simulink model "nonop_quadcopter_package_delivery"  (R2024b)
settings: Solver=VariableStepAuto  StartTime=0.0  StopTime=timespot_spl(end)+2  FixedStep=0.01  MaxStep=1e-2  RelTol=1e-3  AbsTol=1e-3
model workspace (MATLAB code in the model file):
  | load('xy_data_membrane.mat');
undefined symbols (not defined in the file): air_rho, battery_capacity, drone_leg, filtD_altitude, filtD_attitude, filtD_motor, filtD_position, filtD_yaw, filtM_altitude, filtM_attitude, filtM_position, filtM_yaw, filtSpd_motor, kd_altitude, kd_attitude, kd_motor, kd_position, kd_yaw, ki_altitude, ki_attitude, ki_motor, ki_position, ki_yaw, kp_altitude, kp_attitude, kp_motor, kp_position, kp_yaw, limit_altitude, limit_attitude, limit_motor, limit_yaw, planedepth, pos2attitude, propeller, qc_motor, qd_area, qd_drag, spline_data, spline_yaw, timespot_spl, waypoints, wind_speed, X, Y, Z
libraries: sm_lib x73, fl_lib x49, nesl_utility x41, slpidlib x9, batt_lib x4, BatteryEstimators x4, ee_lib x4, quadcopter_library x4, batteryecm_lib x1
(part 4 of 5)

== system nonop_quadcopter_package_delivery/Quadcopter/Electrical/Control2 ==
  ref : Inport
  meas : Inport  Port=2
  Add : Sum  Inputs=+-
  Control : slpidlib/PID Controller  Controller=PID  Form=Parallel  TimeDomain=Continuous-time  UseExternalTs=off  SampleTime=-1  IntegratorMethod=Forward Euler  FilterMethod=Forward Euler  ControllerParametersSource=internal  P=kp  I=ki  UseKiTs=off  D=kd  UseExternalDerivativeSource=off  N=f_deriv  UseFilter=on  TunerSelectOption=Transfer Function Based (PID Tuner App)  ZeroCross=off  InitialConditionSource=internal  InitialConditionForIntegrator=0  InitialConditionForFilter=0  DifferentiatorICPrevScaledInput=0  ExternalReset=none  TrackingMode=off  Kt=1  LimitOutput=on  SatLimitsSource=internal  UpperSaturationLimit=max_trq_cmd  LowerSaturationLimit=-max_trq_cmd  LinearizeAsGain=on  AntiWindupMode=clamping  Kb=1  LimitIntegrator=off  UpperIntegratorSaturationLimit=inf  LowerIntegratorSaturationLimit=-inf  POutMin=[]  POutMax=[]  IOutMin=[]  IOutMax=[]  DOutMin=[]  DOutMax=[]  NOutMin=[]  NOutMax=[]  SumOutMin=[]  SumOutMax=[]  SaturationOutMin=[]  SaturationOutMax=[]  PParamMin=[]  PParamMax=[]  IParamMin=[]  IParamMax=[]  DParamMin=[]  DParamMax=[]  NParamMin=[]  NParamMax=[]  KbParamMin=[]  KbParamMax=[]  KtParamMin=[]  KtParamMax=[]  KbOutMin=[]  KbOutMax=[]  KtOutMin=[]  KtOutMax=[]  IntegratorOutMin=[]  IntegratorOutMax=[]  FilterOutMin=[]  FilterOutMax=[]  SumI1OutMin=[]  SumI1OutMax=[]  SumI2OutMin=[]  SumI2OutMax=[]  SumI3OutMin=[]  SumI3OutMax=[]  SumI4OutMin=[]  SumI4OutMax=[]  SumDOutMin=[]  SumDOutMax=[]  DifferentiatorOutMin=[]  DifferentiatorOutMax=[]  FilterDiffOutCoefMin=[]  FilterDiffOutCoefMax=[]  ReciprocalOutMin=[]  ReciprocalOutMax=[]  SumDenOutMin=[]  SumDenOutMax=[]  SumNumOutMin=[]  SumNumOutMax=[]  DivideOutMin=[]  DivideOutMax=[]  UdiffTsProdOutMin=[]  UdiffTsProdOutMax=[]  NTsProdOutMin=[]  NTsProdOutMax=[]  UintegralTsProdOutMin=[]  UintegralTsProdOutMax=[]  UngainTsProdOutMin=[]  UngainTsProdOutMax=[]  ClampingZeroOutDataTypeStr=Inherit: Inherit via back propagation  ClampingZeroOutMin=[]  ClampingZeroOutMax=[]  FilterDenConstantOutDataTypeStr=Inherit: Inherit via back propagation  FilterDenConstantOutMin=[]  FilterDenConstantOutMax=[]  PCopyOutDataTypeStr=Inherit: Inherit via back propagation  PCopyOutMin=[]  PCopyOutMax=[]  NCopyOutDataTypeStr=Inherit: Inherit via back propagation  NCopyOutMin=[]  NCopyOutMax=[]  IntegratorContinuousStateAttributes=''  IntegratorStateMustResolveToSignalObject=off  IntegratorRTWStateStorageClass=Auto  FilterContinuousStateAttributes=''  FilterStateMustResolveToSignalObject=off  FilterRTWStateStorageClass=Auto  ParallelPVariant=InternalParameters  IdealPVariant=Disabled  IVariant=InternalParameters  DVariant=InternalParameters  IntegratorVariant=Continuous  SatVariant=Enabled  AWVariant=ContClampingParallel  PCopyVariant=Disabled  TRVariant=Disabled  FdbkBlocksVariant=Forward  IdealPFdbkVariant=Disabled  SatFdbkVariant=Disabled  DerivativeFilterVariant=ContFilter  NVariant=InternalParameters  NCopyVariant=Disabled  FilterICVariant=InternalICsFilter  IntegratorICVariant=InternalICs  ExternalResetVariant=Disabled  TRSumVariant=Passthrough  SumFdbkVariant=Disabled  SumVariant=Sum_PID  TsampFilterVariant=InternalTs  TsampNgainVariant=Passthrough  TsampIntegralVariant=Disabled_SignalSpec  ExternalSaturationOutDataTypeStr=Inherit: Same as second input  DerivativeSourceVariant=ErrorSignal  PreIntVariant=InternalPreInt
  Mux : Mux  Inputs=2
  Scope : Scope  NumInputPorts=3
  Transfer Fcn1 : TransferFcn  Denominator=[f_spd 1]
  torque : Outport
  wires:
  Control/1 -> torque/1, Scope/3  "torque"
  ref/1 -> Add/1, Mux/1
  Add/1 -> Scope/2, Control/1  "error"
  Mux/1 -> Scope/1
  meas/1 -> Transfer Fcn1/1
  Transfer Fcn1/1 -> Add/2, Mux/2

== system nonop_quadcopter_package_delivery/Quadcopter/Electrical/Control3 ==
  ref : Inport
  meas : Inport  Port=2
  Add : Sum  Inputs=+-
  Control : slpidlib/PID Controller  Controller=PID  Form=Parallel  TimeDomain=Continuous-time  UseExternalTs=off  SampleTime=-1  IntegratorMethod=Forward Euler  FilterMethod=Forward Euler  ControllerParametersSource=internal  P=kp  I=ki  UseKiTs=off  D=kd  UseExternalDerivativeSource=off  N=f_deriv  UseFilter=on  TunerSelectOption=Transfer Function Based (PID Tuner App)  ZeroCross=off  InitialConditionSource=internal  InitialConditionForIntegrator=0  InitialConditionForFilter=0  DifferentiatorICPrevScaledInput=0  ExternalReset=none  TrackingMode=off  Kt=1  LimitOutput=on  SatLimitsSource=internal  UpperSaturationLimit=max_trq_cmd  LowerSaturationLimit=-max_trq_cmd  LinearizeAsGain=on  AntiWindupMode=clamping  Kb=1  LimitIntegrator=off  UpperIntegratorSaturationLimit=inf  LowerIntegratorSaturationLimit=-inf  POutMin=[]  POutMax=[]  IOutMin=[]  IOutMax=[]  DOutMin=[]  DOutMax=[]  NOutMin=[]  NOutMax=[]  SumOutMin=[]  SumOutMax=[]  SaturationOutMin=[]  SaturationOutMax=[]  PParamMin=[]  PParamMax=[]  IParamMin=[]  IParamMax=[]  DParamMin=[]  DParamMax=[]  NParamMin=[]  NParamMax=[]  KbParamMin=[]  KbParamMax=[]  KtParamMin=[]  KtParamMax=[]  KbOutMin=[]  KbOutMax=[]  KtOutMin=[]  KtOutMax=[]  IntegratorOutMin=[]  IntegratorOutMax=[]  FilterOutMin=[]  FilterOutMax=[]  SumI1OutMin=[]  SumI1OutMax=[]  SumI2OutMin=[]  SumI2OutMax=[]  SumI3OutMin=[]  SumI3OutMax=[]  SumI4OutMin=[]  SumI4OutMax=[]  SumDOutMin=[]  SumDOutMax=[]  DifferentiatorOutMin=[]  DifferentiatorOutMax=[]  FilterDiffOutCoefMin=[]  FilterDiffOutCoefMax=[]  ReciprocalOutMin=[]  ReciprocalOutMax=[]  SumDenOutMin=[]  SumDenOutMax=[]  SumNumOutMin=[]  SumNumOutMax=[]  DivideOutMin=[]  DivideOutMax=[]  UdiffTsProdOutMin=[]  UdiffTsProdOutMax=[]  NTsProdOutMin=[]  NTsProdOutMax=[]  UintegralTsProdOutMin=[]  UintegralTsProdOutMax=[]  UngainTsProdOutMin=[]  UngainTsProdOutMax=[]  ClampingZeroOutDataTypeStr=Inherit: Inherit via back propagation  ClampingZeroOutMin=[]  ClampingZeroOutMax=[]  FilterDenConstantOutDataTypeStr=Inherit: Inherit via back propagation  FilterDenConstantOutMin=[]  FilterDenConstantOutMax=[]  PCopyOutDataTypeStr=Inherit: Inherit via back propagation  PCopyOutMin=[]  PCopyOutMax=[]  NCopyOutDataTypeStr=Inherit: Inherit via back propagation  NCopyOutMin=[]  NCopyOutMax=[]  IntegratorContinuousStateAttributes=''  IntegratorStateMustResolveToSignalObject=off  IntegratorRTWStateStorageClass=Auto  FilterContinuousStateAttributes=''  FilterStateMustResolveToSignalObject=off  FilterRTWStateStorageClass=Auto  ParallelPVariant=InternalParameters  IdealPVariant=Disabled  IVariant=InternalParameters  DVariant=InternalParameters  IntegratorVariant=Continuous  SatVariant=Enabled  AWVariant=ContClampingParallel  PCopyVariant=Disabled  TRVariant=Disabled  FdbkBlocksVariant=Forward  IdealPFdbkVariant=Disabled  SatFdbkVariant=Disabled  DerivativeFilterVariant=ContFilter  NVariant=InternalParameters  NCopyVariant=Disabled  FilterICVariant=InternalICsFilter  IntegratorICVariant=InternalICs  ExternalResetVariant=Disabled  TRSumVariant=Passthrough  SumFdbkVariant=Disabled  SumVariant=Sum_PID  TsampFilterVariant=InternalTs  TsampNgainVariant=Passthrough  TsampIntegralVariant=Disabled_SignalSpec  ExternalSaturationOutDataTypeStr=Inherit: Same as second input  DerivativeSourceVariant=ErrorSignal  PreIntVariant=InternalPreInt
  Mux : Mux  Inputs=2
  Scope : Scope  NumInputPorts=3
  Transfer Fcn1 : TransferFcn  Denominator=[f_spd 1]
  torque : Outport
  wires:
  Control/1 -> torque/1, Scope/3  "torque"
  ref/1 -> Add/1, Mux/1
  Add/1 -> Scope/2, Control/1  "error"
  Mux/1 -> Scope/1
  meas/1 -> Transfer Fcn1/1
  Transfer Fcn1/1 -> Add/2, Mux/2

== system nonop_quadcopter_package_delivery/Quadcopter/Electrical/Control4 ==
  ref : Inport
  meas : Inport  Port=2
  Add : Sum  Inputs=+-
  Control : slpidlib/PID Controller  Controller=PID  Form=Parallel  TimeDomain=Continuous-time  UseExternalTs=off  SampleTime=-1  IntegratorMethod=Forward Euler  FilterMethod=Forward Euler  ControllerParametersSource=internal  P=kp  I=ki  UseKiTs=off  D=kd  UseExternalDerivativeSource=off  N=f_deriv  UseFilter=on  TunerSelectOption=Transfer Function Based (PID Tuner App)  ZeroCross=off  InitialConditionSource=internal  InitialConditionForIntegrator=0  InitialConditionForFilter=0  DifferentiatorICPrevScaledInput=0  ExternalReset=none  TrackingMode=off  Kt=1  LimitOutput=on  SatLimitsSource=internal  UpperSaturationLimit=max_trq_cmd  LowerSaturationLimit=-max_trq_cmd  LinearizeAsGain=on  AntiWindupMode=clamping  Kb=1  LimitIntegrator=off  UpperIntegratorSaturationLimit=inf  LowerIntegratorSaturationLimit=-inf  POutMin=[]  POutMax=[]  IOutMin=[]  IOutMax=[]  DOutMin=[]  DOutMax=[]  NOutMin=[]  NOutMax=[]  SumOutMin=[]  SumOutMax=[]  SaturationOutMin=[]  SaturationOutMax=[]  PParamMin=[]  PParamMax=[]  IParamMin=[]  IParamMax=[]  DParamMin=[]  DParamMax=[]  NParamMin=[]  NParamMax=[]  KbParamMin=[]  KbParamMax=[]  KtParamMin=[]  KtParamMax=[]  KbOutMin=[]  KbOutMax=[]  KtOutMin=[]  KtOutMax=[]  IntegratorOutMin=[]  IntegratorOutMax=[]  FilterOutMin=[]  FilterOutMax=[]  SumI1OutMin=[]  SumI1OutMax=[]  SumI2OutMin=[]  SumI2OutMax=[]  SumI3OutMin=[]  SumI3OutMax=[]  SumI4OutMin=[]  SumI4OutMax=[]  SumDOutMin=[]  SumDOutMax=[]  DifferentiatorOutMin=[]  DifferentiatorOutMax=[]  FilterDiffOutCoefMin=[]  FilterDiffOutCoefMax=[]  ReciprocalOutMin=[]  ReciprocalOutMax=[]  SumDenOutMin=[]  SumDenOutMax=[]  SumNumOutMin=[]  SumNumOutMax=[]  DivideOutMin=[]  DivideOutMax=[]  UdiffTsProdOutMin=[]  UdiffTsProdOutMax=[]  NTsProdOutMin=[]  NTsProdOutMax=[]  UintegralTsProdOutMin=[]  UintegralTsProdOutMax=[]  UngainTsProdOutMin=[]  UngainTsProdOutMax=[]  ClampingZeroOutDataTypeStr=Inherit: Inherit via back propagation  ClampingZeroOutMin=[]  ClampingZeroOutMax=[]  FilterDenConstantOutDataTypeStr=Inherit: Inherit via back propagation  FilterDenConstantOutMin=[]  FilterDenConstantOutMax=[]  PCopyOutDataTypeStr=Inherit: Inherit via back propagation  PCopyOutMin=[]  PCopyOutMax=[]  NCopyOutDataTypeStr=Inherit: Inherit via back propagation  NCopyOutMin=[]  NCopyOutMax=[]  IntegratorContinuousStateAttributes=''  IntegratorStateMustResolveToSignalObject=off  IntegratorRTWStateStorageClass=Auto  FilterContinuousStateAttributes=''  FilterStateMustResolveToSignalObject=off  FilterRTWStateStorageClass=Auto  ParallelPVariant=InternalParameters  IdealPVariant=Disabled  IVariant=InternalParameters  DVariant=InternalParameters  IntegratorVariant=Continuous  SatVariant=Enabled  AWVariant=ContClampingParallel  PCopyVariant=Disabled  TRVariant=Disabled  FdbkBlocksVariant=Forward  IdealPFdbkVariant=Disabled  SatFdbkVariant=Disabled  DerivativeFilterVariant=ContFilter  NVariant=InternalParameters  NCopyVariant=Disabled  FilterICVariant=InternalICsFilter  IntegratorICVariant=InternalICs  ExternalResetVariant=Disabled  TRSumVariant=Passthrough  SumFdbkVariant=Disabled  SumVariant=Sum_PID  TsampFilterVariant=InternalTs  TsampNgainVariant=Passthrough  TsampIntegralVariant=Disabled_SignalSpec  ExternalSaturationOutDataTypeStr=Inherit: Same as second input  DerivativeSourceVariant=ErrorSignal  PreIntVariant=InternalPreInt
  Mux : Mux  Inputs=2
  Scope : Scope  NumInputPorts=3
  Transfer Fcn1 : TransferFcn  Denominator=[f_spd 1]
  torque : Outport
  wires:
  Control/1 -> torque/1, Scope/3  "torque"
  ref/1 -> Add/1, Mux/1
  Add/1 -> Scope/2, Control/1  "error"
  Mux/1 -> Scope/1
  meas/1 -> Transfer Fcn1/1
  Transfer Fcn1/1 -> Add/2, Mux/2

== system nonop_quadcopter_package_delivery/Quadcopter/Electrical/LFP Single Particle Cell ==
  Battery Single Particle : batt_lib/Cells/Electrochemical/Battery Single Particle  ExtrapolationMethod=simscape.enum.extrapolation.nearest  ThicknessAnode=3.4E-5 m  ElectrolyteLayerCountAnode=10  ThicknessSeparator=2.5E-5 m  ElectrolyteLayerCountSeparator=5  ThicknessCathode=8E-5 m  ElectrolyteLayerCountCathode=10  ElectrodePlateArea=1.5 m^2  ParticleRadiusAnode=5E-6 m  ShellCountAnode=40  ParticleRadiusCathode=5E-6 m  ShellCountCathode=40  ActiveMaterialVolumeFractionAnode=0.58  ActiveMaterialVolumeFractionCathode=0.374  OpenCircuitPotentialAnode=[0.200;0.180;0.160;0.140;0.120;0.110;0.102;0.098;0.094;0.092;0.091;0.090;0.089;0.089;0.088;0.088;0.088;0.088;0.088;0.088;0.088;0.087;0.087;0.087;0.086;0.086;0.085;0.085;0.084;0.084;0.083;0.083;0.082;0.082;0.081;0.081;0.080;0.079;0.078] V  OpenCircuitPotentialCathode=[3.200;3.280;3.340;3.380;3.410;3.420;3.425;3.430;3.432;3.433;3.434;3.435;3.435;3.436;3.436;3.437;3.437;3.438;3.438;3.439;3.439;3.440;3.440;3.441;3.441;3.442;3.442;3.443;3.443;3.444;3.444;3.445;3.446;3.447;3.448;3.449;3.460;3.480;3.500] V  NormalizedStoichiometryBreakpoints=linspace(0.025, 0.975, 39)  MaximumConcentrationAnode=30555 mol/m^3  MaximumStoichiometryAnode=0.811  MinimumStoichiometryAnode=0.0132  MaximumConcentrationCathode=22806 mol/m^3  MaximumStoichiometryCathode=0.74  MinimumStoichiometryCathode=0.035  ActiveMaterialDiffusionCoefficientAnode=3E-15 m^2/s  ActiveMaterialDiffusionCoefficientCathode=1E-15 m^2/s  ConductivityAnode=100 S/m  ConductivityCathode=0.5 S/m  CurrentCollectorResistance=1E-3 Ohm  ElectrolyteVolumeFractionAnode=0.3874  ElectrolyteVolumeFractionSeparator=0.45  ElectrolyteVolumeFractionCathode=0.5725  ElectrolyteConductivity=0.29 S/m  BruggemanExponentAnode=1.5  BruggemanExponentSeparator=1.5  BruggemanExponentCathode=1.5  TransferenceNumber=0.363  ElectrolyteDiffusionCoefficient=2E-10 m^2/s  ChargeTransferRateAnode=1E-9 m^(5/2)/(mol^(1/2)*s)  ChargeTransferRateCathode=1E-11 m^(5/2)/(mol^(1/2)*s)  BatteryThermalMass=150 J/K  ArrheniusReferenceTemperature=298.15 K  ActiveMaterialDiffusionActivationEnergyAnode=39000 J/mol  ActiveMaterialDiffusionActivationEnergyCathode=35000 J/mol  ElectrolyteDiffusionActivationEnergy=26600 J/mol  ConductivityActivationEnergyAnode=3000 J/mol  ConductivityActivationEnergyCathode=3000 J/mol  ElectrolyteConductivityActivationEnergy=11000 J/mol  ChargeTransferActivationEnergyAnode=13000 J/mol  ChargeTransferActivationEnergyCathode=20000 J/mol  batteryCurrent_specify=off  batteryCurrent_priority=None  batteryCurrent=0 A  batteryCurrent_nominal_specify=off  batteryCurrent_nominal_value=1  batteryCurrent_nominal_unit=A  batteryVoltage_specify=off  batteryVoltage_priority=None  batteryVoltage=0 V  batteryVoltage_nominal_specify=off  batteryVoltage_nominal_value=1  batteryVoltage_nominal_unit=V  averageElectrolyteConcentration_specify=off  averageElectrolyteConcentration_priority=High  averageElectrolyteConcentration=1200 mol/m^3  averageElectrolyteConcentration_nominal_specify=off  averageElectrolyteConcentration_nominal_value=1  averageElectrolyteConcentration_nominal_unit=mol/m^3  stateOfCharge_specify=off  stateOfCharge_priority=High  stateOfCharge=0.5  stateOfCharge_nominal_specify=off  stateOfCharge_nominal_value=1  stateOfCharge_nominal_unit=1  batteryTemperature_specify=off  batteryTemperature_priority=High  batteryTemperature=298.15 K  batteryTemperature_nominal_specify=off  batteryTemperature_nominal_value=1  batteryTemperature_nominal_unit=K
      settings: InternalSimscapePortConfiguration="{\"Bottom\":[],\"Left\":[{\"id\":\"p\",\"label\":\"+\",\"type\":\"foundation.electrical.electrical\"}],\"Right\":[{\"id\":\"n\",\"label\":\"-\",\"type\":\"foundation.electrical.electrical\"},{\"id\":\"H\",\"label\":\"H\",\"type\":\"foundation.thermal.thermal\"}],\"Top\":[]}"
  Constant : Constant  Value=0.9
  Convective Heat Transfer : fl_lib/Thermal/Thermal Elements/Convective Heat Transfer  thermal_type=foundation.enum.constant_variable.constant  area=0.2 m^2  heat_tr_coeff=15 W/(K*m^2)  min_heat_tr_coeff=1e-3 W/(K*m^2)  T_specify=off  T_priority=None  T=0 K  T_nominal_specify=off  T_nominal_value=1  T_nominal_unit=K  Q_specify=on  Q_priority=None  Q=0 W  Q_nominal_specify=off  Q_nominal_value=1  Q_nominal_unit=W
  Current Sensor : fl_lib/Electrical/Electrical Sensors/Current Sensor
  DC Voltage Source : fl_lib/Electrical/Electrical Sources/DC Voltage Source  v0=15 V
  Electrical Reference : fl_lib/Electrical/Electrical Elements/Electrical Reference
  PS-Sim (I) : nesl_utility/PS-Simulink Converter  PhysicalDomain=network_engine_domain  SubClassName=ps_output  LeftPortType=input  RightPortType=output  PseudoPeriodic=off  Frequencies=[]  VectorFormat=inherit  Unit=A  AffineConversion=off
  PS-Sim (K) : nesl_utility/PS-Simulink Converter  PhysicalDomain=network_engine_domain  SubClassName=ps_output  LeftPortType=input  RightPortType=output  PseudoPeriodic=off  Frequencies=[]  VectorFormat=inherit  Unit=K  AffineConversion=off
  PS-Sim (V) : nesl_utility/PS-Simulink Converter  PhysicalDomain=network_engine_domain  SubClassName=ps_output  LeftPortType=input  RightPortType=output  PseudoPeriodic=off  Frequencies=[]  VectorFormat=inherit  Unit=V  AffineConversion=off
  Rs : fl_lib/Electrical/Electrical Elements/Resistor  R=0.004 Ohm  i_specify=off  i_priority=None  i=0 A  i_nominal_specify=off  i_nominal_value=3  i_nominal_unit=A  v_specify=off  v_priority=None  v=0 V  v_nominal_specify=off  v_nominal_value=3.5  v_nominal_unit=V
  SOC Estimator (Coulomb Counting) : BatteryEstimators/SOC Estimator (Coulomb Counting)  CurrentInputPartition=on  AH=3  Ts=-1
      settings: LibrarySourceBlock=|
      | batt_sl_lib/Estimators/SOC Estimator
      | (Coulomb Counting)
  Temperature Sensor : fl_lib/Thermal/Thermal Sensors/Temperature Sensor  temperature_measure=foundation.enum.MeasurementReference.difference
  Temperature Source : fl_lib/Thermal/Thermal Sources/Temperature Source  temperature=298.15 K
  Thermal Reference : fl_lib/Thermal/Thermal Elements/Thermal Reference
  Voltage Sensor : fl_lib/Electrical/Electrical Sensors/Voltage Sensor
  p : PMIOPort  Side=Left
  n : PMIOPort  Port=2  Side=Right
  SOC : Outport
  Voltage : Outport  Port=2
  Temp : Outport  Port=3
  wires:
  PS-Sim (K)/1 -> Temp/1  "Cell Temperature (K)"
  PS-Sim (I)/1 -> SOC Estimator (Coulomb Counting)/1  "Cell Current (I)"
  PS-Sim (V)/1 -> Voltage/1  "Cell Voltage (V)"
  Constant/1 -> SOC Estimator (Coulomb Counting)/2
  SOC Estimator (Coulomb Counting)/1 -> SOC/1  "Battery State of Charge"
  connections:
  Rs/LConn1 -- Battery Single Particle/LConn1 -- Voltage Sensor/LConn1 -- DC Voltage Source/LConn1
  Battery Single Particle/RConn1 -- DC Voltage Source/RConn1 -- n/RConn1 -- Voltage Sensor/RConn2 -- Electrical Reference/LConn1
  Current Sensor/LConn1 -- p/RConn1
  Convective Heat Transfer/LConn1 -- Battery Single Particle/RConn2 -- Temperature Sensor/LConn1
  Voltage Sensor/RConn1 -- PS-Sim (V)/LConn1
  PS-Sim (I)/LConn1 -- Current Sensor/RConn1
  Current Sensor/RConn2 -- Rs/RConn1
  Thermal Reference/LConn1 -- Temperature Sensor/RConn1
  Temperature Source/LConn1 -- Convective Heat Transfer/RConn1
  Temperature Sensor/RConn2 -- PS-Sim (K)/LConn1

== system nonop_quadcopter_package_delivery/Quadcopter/Electrical/LFP Single Particle Cell1 ==
  Battery Single Particle : batt_lib/Cells/Electrochemical/Battery Single Particle  ExtrapolationMethod=simscape.enum.extrapolation.nearest  ThicknessAnode=3.4E-5 m  ElectrolyteLayerCountAnode=10  ThicknessSeparator=2.5E-5 m  ElectrolyteLayerCountSeparator=5  ThicknessCathode=8E-5 m  ElectrolyteLayerCountCathode=10  ElectrodePlateArea=1.5 m^2  ParticleRadiusAnode=5E-6 m  ShellCountAnode=40  ParticleRadiusCathode=5E-6 m  ShellCountCathode=40  ActiveMaterialVolumeFractionAnode=0.58  ActiveMaterialVolumeFractionCathode=0.374  OpenCircuitPotentialAnode=[0.200;0.180;0.160;0.140;0.120;0.110;0.102;0.098;0.094;0.092;0.091;0.090;0.089;0.089;0.088;0.088;0.088;0.088;0.088;0.088;0.088;0.087;0.087;0.087;0.086;0.086;0.085;0.085;0.084;0.084;0.083;0.083;0.082;0.082;0.081;0.081;0.080;0.079;0.078] V  OpenCircuitPotentialCathode=[3.200;3.280;3.340;3.380;3.410;3.420;3.425;3.430;3.432;3.433;3.434;3.435;3.435;3.436;3.436;3.437;3.437;3.438;3.438;3.439;3.439;3.440;3.440;3.441;3.441;3.442;3.442;3.443;3.443;3.444;3.444;3.445;3.446;3.447;3.448;3.449;3.460;3.480;3.500] V  NormalizedStoichiometryBreakpoints=linspace(0.025, 0.975, 39)  MaximumConcentrationAnode=30555 mol/m^3  MaximumStoichiometryAnode=0.811  MinimumStoichiometryAnode=0.0132  MaximumConcentrationCathode=22806 mol/m^3  MaximumStoichiometryCathode=0.74  MinimumStoichiometryCathode=0.035  ActiveMaterialDiffusionCoefficientAnode=3E-15 m^2/s  ActiveMaterialDiffusionCoefficientCathode=1E-15 m^2/s  ConductivityAnode=100 S/m  ConductivityCathode=0.5 S/m  CurrentCollectorResistance=1E-3 Ohm  ElectrolyteVolumeFractionAnode=0.3874  ElectrolyteVolumeFractionSeparator=0.45  ElectrolyteVolumeFractionCathode=0.5725  ElectrolyteConductivity=0.29 S/m  BruggemanExponentAnode=1.5  BruggemanExponentSeparator=1.5  BruggemanExponentCathode=1.5  TransferenceNumber=0.363  ElectrolyteDiffusionCoefficient=2E-10 m^2/s  ChargeTransferRateAnode=1E-9 m^(5/2)/(mol^(1/2)*s)  ChargeTransferRateCathode=1E-11 m^(5/2)/(mol^(1/2)*s)  BatteryThermalMass=150 J/K  ArrheniusReferenceTemperature=298.15 K  ActiveMaterialDiffusionActivationEnergyAnode=39000 J/mol  ActiveMaterialDiffusionActivationEnergyCathode=35000 J/mol  ElectrolyteDiffusionActivationEnergy=26600 J/mol  ConductivityActivationEnergyAnode=3000 J/mol  ConductivityActivationEnergyCathode=3000 J/mol  ElectrolyteConductivityActivationEnergy=11000 J/mol  ChargeTransferActivationEnergyAnode=13000 J/mol  ChargeTransferActivationEnergyCathode=20000 J/mol  batteryCurrent_specify=off  batteryCurrent_priority=None  batteryCurrent=0 A  batteryCurrent_nominal_specify=off  batteryCurrent_nominal_value=1  batteryCurrent_nominal_unit=A  batteryVoltage_specify=off  batteryVoltage_priority=None  batteryVoltage=0 V  batteryVoltage_nominal_specify=off  batteryVoltage_nominal_value=1  batteryVoltage_nominal_unit=V  averageElectrolyteConcentration_specify=off  averageElectrolyteConcentration_priority=High  averageElectrolyteConcentration=1200 mol/m^3  averageElectrolyteConcentration_nominal_specify=off  averageElectrolyteConcentration_nominal_value=1  averageElectrolyteConcentration_nominal_unit=mol/m^3  stateOfCharge_specify=off  stateOfCharge_priority=High  stateOfCharge=0.5  stateOfCharge_nominal_specify=off  stateOfCharge_nominal_value=1  stateOfCharge_nominal_unit=1  batteryTemperature_specify=off  batteryTemperature_priority=High  batteryTemperature=298.15 K  batteryTemperature_nominal_specify=off  batteryTemperature_nominal_value=1  batteryTemperature_nominal_unit=K
      settings: InternalSimscapePortConfiguration="{\"Bottom\":[],\"Left\":[{\"id\":\"p\",\"label\":\"+\",\"type\":\"foundation.electrical.electrical\"}],\"Right\":[{\"id\":\"n\",\"label\":\"-\",\"type\":\"foundation.electrical.electrical\"},{\"id\":\"H\",\"label\":\"H\",\"type\":\"foundation.thermal.thermal\"}],\"Top\":[]}"
  Constant : Constant  Value=0.9
  Convective Heat Transfer : fl_lib/Thermal/Thermal Elements/Convective Heat Transfer  thermal_type=foundation.enum.constant_variable.constant  area=0.2 m^2  heat_tr_coeff=15 W/(K*m^2)  min_heat_tr_coeff=1e-3 W/(K*m^2)  T_specify=off  T_priority=None  T=0 K  T_nominal_specify=off  T_nominal_value=1  T_nominal_unit=K  Q_specify=on  Q_priority=None  Q=0 W  Q_nominal_specify=off  Q_nominal_value=1  Q_nominal_unit=W
  Current Sensor : fl_lib/Electrical/Electrical Sensors/Current Sensor
  DC Voltage Source : fl_lib/Electrical/Electrical Sources/DC Voltage Source  v0=15 V
  Electrical Reference : fl_lib/Electrical/Electrical Elements/Electrical Reference
  PS-Sim (I) : nesl_utility/PS-Simulink Converter  PhysicalDomain=network_engine_domain  SubClassName=ps_output  LeftPortType=input  RightPortType=output  PseudoPeriodic=off  Frequencies=[]  VectorFormat=inherit  Unit=A  AffineConversion=off
  PS-Sim (K) : nesl_utility/PS-Simulink Converter  PhysicalDomain=network_engine_domain  SubClassName=ps_output  LeftPortType=input  RightPortType=output  PseudoPeriodic=off  Frequencies=[]  VectorFormat=inherit  Unit=K  AffineConversion=off
  PS-Sim (V) : nesl_utility/PS-Simulink Converter  PhysicalDomain=network_engine_domain  SubClassName=ps_output  LeftPortType=input  RightPortType=output  PseudoPeriodic=off  Frequencies=[]  VectorFormat=inherit  Unit=V  AffineConversion=off
  Rs : fl_lib/Electrical/Electrical Elements/Resistor  R=0.004 Ohm  i_specify=off  i_priority=None  i=0 A  i_nominal_specify=off  i_nominal_value=3  i_nominal_unit=A  v_specify=off  v_priority=None  v=0 V  v_nominal_specify=off  v_nominal_value=3.5  v_nominal_unit=V
  SOC Estimator (Coulomb Counting) : BatteryEstimators/SOC Estimator (Coulomb Counting)  CurrentInputPartition=on  AH=3  Ts=-1
      settings: LibrarySourceBlock=|
      | batt_sl_lib/Estimators/SOC Estimator
      | (Coulomb Counting)
  Temperature Sensor : fl_lib/Thermal/Thermal Sensors/Temperature Sensor  temperature_measure=foundation.enum.MeasurementReference.difference
  Temperature Source : fl_lib/Thermal/Thermal Sources/Temperature Source  temperature=298.15 K
  Thermal Reference : fl_lib/Thermal/Thermal Elements/Thermal Reference
  Voltage Sensor : fl_lib/Electrical/Electrical Sensors/Voltage Sensor
  p : PMIOPort  Side=Left
  n : PMIOPort  Port=2  Side=Right
  SOC : Outport
  Voltage : Outport  Port=2
  Temp : Outport  Port=3
  wires:
  PS-Sim (K)/1 -> Temp/1  "Cell Temperature (K)"
  PS-Sim (I)/1 -> SOC Estimator (Coulomb Counting)/1  "Cell Current (I)"
  PS-Sim (V)/1 -> Voltage/1  "Cell Voltage (V)"
  Constant/1 -> SOC Estimator (Coulomb Counting)/2
  SOC Estimator (Coulomb Counting)/1 -> SOC/1  "Battery State of Charge"
  connections:
  Battery Single Particle/LConn1 -- Voltage Sensor/LConn1 -- Rs/LConn1 -- DC Voltage Source/LConn1
  n/RConn1 -- Voltage Sensor/RConn2 -- Electrical Reference/LConn1 -- Battery Single Particle/RConn1 -- DC Voltage Source/RConn1
  Current Sensor/LConn1 -- p/RConn1
  Convective Heat Transfer/LConn1 -- Battery Single Particle/RConn2 -- Temperature Sensor/LConn1
  Voltage Sensor/RConn1 -- PS-Sim (V)/LConn1
  PS-Sim (I)/LConn1 -- Current Sensor/RConn1
  Current Sensor/RConn2 -- Rs/RConn1
  Thermal Reference/LConn1 -- Temperature Sensor/RConn1
  Temperature Source/LConn1 -- Convective Heat Transfer/RConn1
  Temperature Sensor/RConn2 -- PS-Sim (K)/LConn1

== system nonop_quadcopter_package_delivery/Quadcopter/Electrical/LFP Single Particle Cell2 ==
  Battery Single Particle : batt_lib/Cells/Electrochemical/Battery Single Particle  ExtrapolationMethod=simscape.enum.extrapolation.nearest  ThicknessAnode=3.4E-5 m  ElectrolyteLayerCountAnode=10  ThicknessSeparator=2.5E-5 m  ElectrolyteLayerCountSeparator=5  ThicknessCathode=8E-5 m  ElectrolyteLayerCountCathode=10  ElectrodePlateArea=1.5 m^2  ParticleRadiusAnode=5E-6 m  ShellCountAnode=40  ParticleRadiusCathode=5E-6 m  ShellCountCathode=40  ActiveMaterialVolumeFractionAnode=0.58  ActiveMaterialVolumeFractionCathode=0.374  OpenCircuitPotentialAnode=[0.200;0.180;0.160;0.140;0.120;0.110;0.102;0.098;0.094;0.092;0.091;0.090;0.089;0.089;0.088;0.088;0.088;0.088;0.088;0.088;0.088;0.087;0.087;0.087;0.086;0.086;0.085;0.085;0.084;0.084;0.083;0.083;0.082;0.082;0.081;0.081;0.080;0.079;0.078] V  OpenCircuitPotentialCathode=[3.200;3.280;3.340;3.380;3.410;3.420;3.425;3.430;3.432;3.433;3.434;3.435;3.435;3.436;3.436;3.437;3.437;3.438;3.438;3.439;3.439;3.440;3.440;3.441;3.441;3.442;3.442;3.443;3.443;3.444;3.444;3.445;3.446;3.447;3.448;3.449;3.460;3.480;3.500] V  NormalizedStoichiometryBreakpoints=linspace(0.025, 0.975, 39)  MaximumConcentrationAnode=30555 mol/m^3  MaximumStoichiometryAnode=0.811  MinimumStoichiometryAnode=0.0132  MaximumConcentrationCathode=22806 mol/m^3  MaximumStoichiometryCathode=0.74  MinimumStoichiometryCathode=0.035  ActiveMaterialDiffusionCoefficientAnode=3E-15 m^2/s  ActiveMaterialDiffusionCoefficientCathode=1E-15 m^2/s  ConductivityAnode=100 S/m  ConductivityCathode=0.5 S/m  CurrentCollectorResistance=1E-3 Ohm  ElectrolyteVolumeFractionAnode=0.3874  ElectrolyteVolumeFractionSeparator=0.45  ElectrolyteVolumeFractionCathode=0.5725  ElectrolyteConductivity=0.29 S/m  BruggemanExponentAnode=1.5  BruggemanExponentSeparator=1.5  BruggemanExponentCathode=1.5  TransferenceNumber=0.363  ElectrolyteDiffusionCoefficient=2E-10 m^2/s  ChargeTransferRateAnode=1E-9 m^(5/2)/(mol^(1/2)*s)  ChargeTransferRateCathode=1E-11 m^(5/2)/(mol^(1/2)*s)  BatteryThermalMass=150 J/K  ArrheniusReferenceTemperature=298.15 K  ActiveMaterialDiffusionActivationEnergyAnode=39000 J/mol  ActiveMaterialDiffusionActivationEnergyCathode=35000 J/mol  ElectrolyteDiffusionActivationEnergy=26600 J/mol  ConductivityActivationEnergyAnode=3000 J/mol  ConductivityActivationEnergyCathode=3000 J/mol  ElectrolyteConductivityActivationEnergy=11000 J/mol  ChargeTransferActivationEnergyAnode=13000 J/mol  ChargeTransferActivationEnergyCathode=20000 J/mol  batteryCurrent_specify=off  batteryCurrent_priority=None  batteryCurrent=0 A  batteryCurrent_nominal_specify=off  batteryCurrent_nominal_value=1  batteryCurrent_nominal_unit=A  batteryVoltage_specify=off  batteryVoltage_priority=None  batteryVoltage=0 V  batteryVoltage_nominal_specify=off  batteryVoltage_nominal_value=1  batteryVoltage_nominal_unit=V  averageElectrolyteConcentration_specify=off  averageElectrolyteConcentration_priority=High  averageElectrolyteConcentration=1200 mol/m^3  averageElectrolyteConcentration_nominal_specify=off  averageElectrolyteConcentration_nominal_value=1  averageElectrolyteConcentration_nominal_unit=mol/m^3  stateOfCharge_specify=off  stateOfCharge_priority=High  stateOfCharge=0.5  stateOfCharge_nominal_specify=off  stateOfCharge_nominal_value=1  stateOfCharge_nominal_unit=1  batteryTemperature_specify=off  batteryTemperature_priority=High  batteryTemperature=298.15 K  batteryTemperature_nominal_specify=off  batteryTemperature_nominal_value=1  batteryTemperature_nominal_unit=K
      settings: InternalSimscapePortConfiguration="{\"Bottom\":[],\"Left\":[{\"id\":\"p\",\"label\":\"+\",\"type\":\"foundation.electrical.electrical\"}],\"Right\":[{\"id\":\"n\",\"label\":\"-\",\"type\":\"foundation.electrical.electrical\"},{\"id\":\"H\",\"label\":\"H\",\"type\":\"foundation.thermal.thermal\"}],\"Top\":[]}"
  Constant : Constant  Value=0.9
  Convective Heat Transfer : fl_lib/Thermal/Thermal Elements/Convective Heat Transfer  thermal_type=foundation.enum.constant_variable.constant  area=0.2 m^2  heat_tr_coeff=15 W/(K*m^2)  min_heat_tr_coeff=1e-3 W/(K*m^2)  T_specify=off  T_priority=None  T=0 K  T_nominal_specify=off  T_nominal_value=1  T_nominal_unit=K  Q_specify=on  Q_priority=None  Q=0 W  Q_nominal_specify=off  Q_nominal_value=1  Q_nominal_unit=W
  Current Sensor : fl_lib/Electrical/Electrical Sensors/Current Sensor
  DC Voltage Source : fl_lib/Electrical/Electrical Sources/DC Voltage Source  v0=15 V
  Electrical Reference : fl_lib/Electrical/Electrical Elements/Electrical Reference
  PS-Sim (I) : nesl_utility/PS-Simulink Converter  PhysicalDomain=network_engine_domain  SubClassName=ps_output  LeftPortType=input  RightPortType=output  PseudoPeriodic=off  Frequencies=[]  VectorFormat=inherit  Unit=A  AffineConversion=off
  PS-Sim (K) : nesl_utility/PS-Simulink Converter  PhysicalDomain=network_engine_domain  SubClassName=ps_output  LeftPortType=input  RightPortType=output  PseudoPeriodic=off  Frequencies=[]  VectorFormat=inherit  Unit=K  AffineConversion=off
  PS-Sim (V) : nesl_utility/PS-Simulink Converter  PhysicalDomain=network_engine_domain  SubClassName=ps_output  LeftPortType=input  RightPortType=output  PseudoPeriodic=off  Frequencies=[]  VectorFormat=inherit  Unit=V  AffineConversion=off
  Rs : fl_lib/Electrical/Electrical Elements/Resistor  R=0.004 Ohm  i_specify=off  i_priority=None  i=0 A  i_nominal_specify=off  i_nominal_value=3  i_nominal_unit=A  v_specify=off  v_priority=None  v=0 V  v_nominal_specify=off  v_nominal_value=3.5  v_nominal_unit=V
  SOC Estimator (Coulomb Counting) : BatteryEstimators/SOC Estimator (Coulomb Counting)  CurrentInputPartition=on  AH=3  Ts=-1
      settings: LibrarySourceBlock=|
      | batt_sl_lib/Estimators/SOC Estimator
      | (Coulomb Counting)
  Temperature Sensor : fl_lib/Thermal/Thermal Sensors/Temperature Sensor  temperature_measure=foundation.enum.MeasurementReference.difference
  Temperature Source : fl_lib/Thermal/Thermal Sources/Temperature Source  temperature=298.15 K
  Thermal Reference : fl_lib/Thermal/Thermal Elements/Thermal Reference
  Voltage Sensor : fl_lib/Electrical/Electrical Sensors/Voltage Sensor
  p : PMIOPort  Side=Left
  n : PMIOPort  Port=2  Side=Right
  SOC : Outport
  Voltage : Outport  Port=2
  Temp : Outport  Port=3
  wires:
  PS-Sim (K)/1 -> Temp/1  "Cell Temperature (K)"
  PS-Sim (I)/1 -> SOC Estimator (Coulomb Counting)/1  "Cell Current (I)"
  PS-Sim (V)/1 -> Voltage/1  "Cell Voltage (V)"
  Constant/1 -> SOC Estimator (Coulomb Counting)/2
  SOC Estimator (Coulomb Counting)/1 -> SOC/1  "Battery State of Charge"
  connections:
  Battery Single Particle/LConn1 -- Voltage Sensor/LConn1 -- Rs/LConn1 -- DC Voltage Source/LConn1
  n/RConn1 -- Voltage Sensor/RConn2 -- Electrical Reference/LConn1 -- Battery Single Particle/RConn1 -- DC Voltage Source/RConn1
  Current Sensor/LConn1 -- p/RConn1
  Convective Heat Transfer/LConn1 -- Battery Single Particle/RConn2 -- Temperature Sensor/LConn1
  Voltage Sensor/RConn1 -- PS-Sim (V)/LConn1
  PS-Sim (I)/LConn1 -- Current Sensor/RConn1
  Current Sensor/RConn2 -- Rs/RConn1
  Thermal Reference/LConn1 -- Temperature Sensor/RConn1
  Temperature Source/LConn1 -- Convective Heat Transfer/RConn1
  Temperature Sensor/RConn2 -- PS-Sim (K)/LConn1

== system nonop_quadcopter_package_delivery/Quadcopter/Electrical/LFP Single Particle Cell3 ==
  Battery Single Particle : batt_lib/Cells/Electrochemical/Battery Single Particle  ExtrapolationMethod=simscape.enum.extrapolation.nearest  ThicknessAnode=3.4E-5 m  ElectrolyteLayerCountAnode=10  ThicknessSeparator=2.5E-5 m  ElectrolyteLayerCountSeparator=5  ThicknessCathode=8E-5 m  ElectrolyteLayerCountCathode=10  ElectrodePlateArea=1.5 m^2  ParticleRadiusAnode=5E-6 m  ShellCountAnode=40  ParticleRadiusCathode=5E-6 m  ShellCountCathode=40  ActiveMaterialVolumeFractionAnode=0.58  ActiveMaterialVolumeFractionCathode=0.374  OpenCircuitPotentialAnode=[0.200;0.180;0.160;0.140;0.120;0.110;0.102;0.098;0.094;0.092;0.091;0.090;0.089;0.089;0.088;0.088;0.088;0.088;0.088;0.088;0.088;0.087;0.087;0.087;0.086;0.086;0.085;0.085;0.084;0.084;0.083;0.083;0.082;0.082;0.081;0.081;0.080;0.079;0.078] V  OpenCircuitPotentialCathode=[3.200;3.280;3.340;3.380;3.410;3.420;3.425;3.430;3.432;3.433;3.434;3.435;3.435;3.436;3.436;3.437;3.437;3.438;3.438;3.439;3.439;3.440;3.440;3.441;3.441;3.442;3.442;3.443;3.443;3.444;3.444;3.445;3.446;3.447;3.448;3.449;3.460;3.480;3.500] V  NormalizedStoichiometryBreakpoints=linspace(0.025, 0.975, 39)  MaximumConcentrationAnode=30555 mol/m^3  MaximumStoichiometryAnode=0.811  MinimumStoichiometryAnode=0.0132  MaximumConcentrationCathode=22806 mol/m^3  MaximumStoichiometryCathode=0.74  MinimumStoichiometryCathode=0.035  ActiveMaterialDiffusionCoefficientAnode=3E-15 m^2/s  ActiveMaterialDiffusionCoefficientCathode=1E-15 m^2/s  ConductivityAnode=100 S/m  ConductivityCathode=0.5 S/m  CurrentCollectorResistance=1E-3 Ohm  ElectrolyteVolumeFractionAnode=0.3874  ElectrolyteVolumeFractionSeparator=0.45  ElectrolyteVolumeFractionCathode=0.5725  ElectrolyteConductivity=0.29 S/m  BruggemanExponentAnode=1.5  BruggemanExponentSeparator=1.5  BruggemanExponentCathode=1.5  TransferenceNumber=0.363  ElectrolyteDiffusionCoefficient=2E-10 m^2/s  ChargeTransferRateAnode=1E-9 m^(5/2)/(mol^(1/2)*s)  ChargeTransferRateCathode=1E-11 m^(5/2)/(mol^(1/2)*s)  BatteryThermalMass=150 J/K  ArrheniusReferenceTemperature=298.15 K  ActiveMaterialDiffusionActivationEnergyAnode=39000 J/mol  ActiveMaterialDiffusionActivationEnergyCathode=35000 J/mol  ElectrolyteDiffusionActivationEnergy=26600 J/mol  ConductivityActivationEnergyAnode=3000 J/mol  ConductivityActivationEnergyCathode=3000 J/mol  ElectrolyteConductivityActivationEnergy=11000 J/mol  ChargeTransferActivationEnergyAnode=13000 J/mol  ChargeTransferActivationEnergyCathode=20000 J/mol  batteryCurrent_specify=off  batteryCurrent_priority=None  batteryCurrent=0 A  batteryCurrent_nominal_specify=off  batteryCurrent_nominal_value=1  batteryCurrent_nominal_unit=A  batteryVoltage_specify=off  batteryVoltage_priority=None  batteryVoltage=0 V  batteryVoltage_nominal_specify=off  batteryVoltage_nominal_value=1  batteryVoltage_nominal_unit=V  averageElectrolyteConcentration_specify=off  averageElectrolyteConcentration_priority=High  averageElectrolyteConcentration=1200 mol/m^3  averageElectrolyteConcentration_nominal_specify=off  averageElectrolyteConcentration_nominal_value=1  averageElectrolyteConcentration_nominal_unit=mol/m^3  stateOfCharge_specify=off  stateOfCharge_priority=High  stateOfCharge=0.5  stateOfCharge_nominal_specify=off  stateOfCharge_nominal_value=1  stateOfCharge_nominal_unit=1  batteryTemperature_specify=off  batteryTemperature_priority=High  batteryTemperature=298.15 K  batteryTemperature_nominal_specify=off  batteryTemperature_nominal_value=1  batteryTemperature_nominal_unit=K
      settings: InternalSimscapePortConfiguration="{\"Bottom\":[],\"Left\":[{\"id\":\"p\",\"label\":\"+\",\"type\":\"foundation.electrical.electrical\"}],\"Right\":[{\"id\":\"n\",\"label\":\"-\",\"type\":\"foundation.electrical.electrical\"},{\"id\":\"H\",\"label\":\"H\",\"type\":\"foundation.thermal.thermal\"}],\"Top\":[]}"
  Constant : Constant  Value=0.9
  Convective Heat Transfer : fl_lib/Thermal/Thermal Elements/Convective Heat Transfer  thermal_type=foundation.enum.constant_variable.constant  area=0.2 m^2  heat_tr_coeff=15 W/(K*m^2)  min_heat_tr_coeff=1e-3 W/(K*m^2)  T_specify=off  T_priority=None  T=0 K  T_nominal_specify=off  T_nominal_value=1  T_nominal_unit=K  Q_specify=on  Q_priority=None  Q=0 W  Q_nominal_specify=off  Q_nominal_value=1  Q_nominal_unit=W
  Current Sensor : fl_lib/Electrical/Electrical Sensors/Current Sensor
  DC Voltage Source : fl_lib/Electrical/Electrical Sources/DC Voltage Source  v0=15 V
  Electrical Reference : fl_lib/Electrical/Electrical Elements/Electrical Reference
  PS-Sim (I) : nesl_utility/PS-Simulink Converter  PhysicalDomain=network_engine_domain  SubClassName=ps_output  LeftPortType=input  RightPortType=output  PseudoPeriodic=off  Frequencies=[]  VectorFormat=inherit  Unit=A  AffineConversion=off
  PS-Sim (K) : nesl_utility/PS-Simulink Converter  PhysicalDomain=network_engine_domain  SubClassName=ps_output  LeftPortType=input  RightPortType=output  PseudoPeriodic=off  Frequencies=[]  VectorFormat=inherit  Unit=K  AffineConversion=off
  PS-Sim (V) : nesl_utility/PS-Simulink Converter  PhysicalDomain=network_engine_domain  SubClassName=ps_output  LeftPortType=input  RightPortType=output  PseudoPeriodic=off  Frequencies=[]  VectorFormat=inherit  Unit=V  AffineConversion=off
  Rs : fl_lib/Electrical/Electrical Elements/Resistor  R=0.004 Ohm  i_specify=off  i_priority=None  i=0 A  i_nominal_specify=off  i_nominal_value=3  i_nominal_unit=A  v_specify=off  v_priority=None  v=0 V  v_nominal_specify=off  v_nominal_value=3.5  v_nominal_unit=V
  SOC Estimator (Coulomb Counting) : BatteryEstimators/SOC Estimator (Coulomb Counting)  CurrentInputPartition=on  AH=3  Ts=-1
      settings: LibrarySourceBlock=|
      | batt_sl_lib/Estimators/SOC Estimator
      | (Coulomb Counting)
  Temperature Sensor : fl_lib/Thermal/Thermal Sensors/Temperature Sensor  temperature_measure=foundation.enum.MeasurementReference.difference
  Temperature Source : fl_lib/Thermal/Thermal Sources/Temperature Source  temperature=298.15 K
  Thermal Reference : fl_lib/Thermal/Thermal Elements/Thermal Reference
  Voltage Sensor : fl_lib/Electrical/Electrical Sensors/Voltage Sensor
  p : PMIOPort  Side=Left
  n : PMIOPort  Port=2  Side=Right
  SOC : Outport
  Voltage : Outport  Port=2
  Temp : Outport  Port=3
  wires:
  PS-Sim (K)/1 -> Temp/1  "Cell Temperature (K)"
  PS-Sim (I)/1 -> SOC Estimator (Coulomb Counting)/1  "Cell Current (I)"
  PS-Sim (V)/1 -> Voltage/1  "Cell Voltage (V)"
  Constant/1 -> SOC Estimator (Coulomb Counting)/2
  SOC Estimator (Coulomb Counting)/1 -> SOC/1  "Battery State of Charge"
  connections:
  Battery Single Particle/LConn1 -- Voltage Sensor/LConn1 -- Rs/LConn1 -- DC Voltage Source/LConn1
  n/RConn1 -- Voltage Sensor/RConn2 -- Electrical Reference/LConn1 -- Battery Single Particle/RConn1 -- DC Voltage Source/RConn1
  Current Sensor/LConn1 -- p/RConn1
  Convective Heat Transfer/LConn1 -- Battery Single Particle/RConn2 -- Temperature Sensor/LConn1
  Voltage Sensor/RConn1 -- PS-Sim (V)/LConn1
  PS-Sim (I)/LConn1 -- Current Sensor/RConn1
  Current Sensor/RConn2 -- Rs/RConn1
  Thermal Reference/LConn1 -- Temperature Sensor/RConn1
  Temperature Source/LConn1 -- Convective Heat Transfer/RConn1
  Temperature Sensor/RConn2 -- PS-Sim (K)/LConn1

== system nonop_quadcopter_package_delivery/Quadcopter/Electrical/Sensing Temperature ==
  PS-Simulink Converter : nesl_utility/PS-Simulink Converter  PhysicalDomain=network_engine_domain  SubClassName=ps_output  LeftPortType=input  RightPortType=output  PseudoPeriodic=off  Frequencies=[]  VectorFormat=1-D array  Unit=inherit  AffineConversion=off
  Temperature Sensor : fl_lib/Thermal/Thermal Sensors/Temperature Sensor  temperature_measure=foundation.enum.MeasurementReference.difference
  Thermal Reference : fl_lib/Thermal/Thermal Elements/Thermal Reference
  A : PMIOPort  Side=Left
  T : Outport
  wires:
  PS-Simulink Converter/1 -> T/1
  connections:
  Thermal Reference/LConn1 -- Temperature Sensor/RConn1
  Temperature Sensor/RConn2 -- PS-Simulink Converter/LConn1
  A/RConn1 -- Temperature Sensor/LConn1

== system nonop_quadcopter_package_delivery/Quadcopter/Electrical/Sensor M1 ==
  Current Sensor : fl_lib/Electrical/Electrical Sensors/Current Sensor
  PS-Simulink Converter3 : nesl_utility/PS-Simulink Converter  PhysicalDomain=network_engine_domain  SubClassName=ps_output  LeftPortType=input  RightPortType=output  PseudoPeriodic=off  Frequencies=[]  VectorFormat=1-D array  Unit=inherit  AffineConversion=off
  + : PMIOPort  Side=Left
  - : PMIOPort  Port=2  Side=Right
  i : Outport
  wires:
  PS-Simulink Converter3/1 -> i/1
  connections:
  +/RConn1 -- Current Sensor/LConn1
  Current Sensor/RConn2 -- -/RConn1
  PS-Simulink Converter3/LConn1 -- Current Sensor/RConn1

== system nonop_quadcopter_package_delivery/Quadcopter/Electrical/Sensor M2 ==
  Current Sensor : fl_lib/Electrical/Electrical Sensors/Current Sensor
  PS-Simulink Converter3 : nesl_utility/PS-Simulink Converter  PhysicalDomain=network_engine_domain  SubClassName=ps_output  LeftPortType=input  RightPortType=output  PseudoPeriodic=off  Frequencies=[]  VectorFormat=1-D array  Unit=inherit  AffineConversion=off
  + : PMIOPort  Side=Left
  - : PMIOPort  Port=2  Side=Right
  i : Outport
  wires:
  PS-Simulink Converter3/1 -> i/1
  connections:
  PS-Simulink Converter3/LConn1 -- Current Sensor/RConn1
  Current Sensor/RConn2 -- -/RConn1
  +/RConn1 -- Current Sensor/LConn1

== system nonop_quadcopter_package_delivery/Quadcopter/Electrical/Sensor M3 ==
  Current Sensor : fl_lib/Electrical/Electrical Sensors/Current Sensor
  PS-Simulink Converter3 : nesl_utility/PS-Simulink Converter  PhysicalDomain=network_engine_domain  SubClassName=ps_output  LeftPortType=input  RightPortType=output  PseudoPeriodic=off  Frequencies=[]  VectorFormat=1-D array  Unit=inherit  AffineConversion=off
  + : PMIOPort  Side=Left
  - : PMIOPort  Port=2  Side=Right
  i : Outport
  wires:
  PS-Simulink Converter3/1 -> i/1
  connections:
  +/RConn1 -- Current Sensor/LConn1
  Current Sensor/RConn2 -- -/RConn1
  PS-Simulink Converter3/LConn1 -- Current Sensor/RConn1

== system nonop_quadcopter_package_delivery/Quadcopter/Electrical/Sensor M4 ==
  Current Sensor : fl_lib/Electrical/Electrical Sensors/Current Sensor
  PS-Simulink Converter3 : nesl_utility/PS-Simulink Converter  PhysicalDomain=network_engine_domain  SubClassName=ps_output  LeftPortType=input  RightPortType=output  PseudoPeriodic=off  Frequencies=[]  VectorFormat=1-D array  Unit=inherit  AffineConversion=off
  + : PMIOPort  Side=Left
  - : PMIOPort  Port=2  Side=Right
  i : Outport
  wires:
  PS-Simulink Converter3/1 -> i/1
  connections:
  PS-Simulink Converter3/LConn1 -- Current Sensor/RConn1
  Current Sensor/RConn2 -- -/RConn1
  +/RConn1 -- Current Sensor/LConn1

== system nonop_quadcopter_package_delivery/Quadcopter/Ground/Ground ==
  Ground : sm_lib/Body Elements/Brick Solid  BrickDimensions=[plane_x plane_y planedepth]  BrickDimensionsUnits=m  ExportEntireGeometry=off  InertiaType=CalculateFromGeometry  BasedOnType=Density  Density=1000  DensityUnits=kg/m^3  Mass=1  MassUnits=kg  CenterOfMass=[0 0 0]  CenterOfMassUnits=m  MomentsOfInertia=[1 1 1]  MomentsOfInertiaUnits=kg*m^2  ProductsOfInertia=[0 0 0]  ProductsOfInertiaUnits=kg*m^2  GraphicType=FromGeometry  MarkerShape=Sphere  MarkerSize=10  GraphicVisPropType=SimpleVisualProperties  GraphicDiffuseColor=[0.0 0.7 0.1]  GraphicOpacity=1  GraphicSpecularColor=[0.5 0.5 0.5 1.0]  GraphicAmbientColor=[0.15 0.15 0.15 1.0]  GraphicEmissiveColor=[0.0 0.0 0.0 1.0]  GraphicShininess=75  DoExposeReferenceFrame=on  SerializedFrames=<Frames><Frame><Id>Frame1</Id><Value><Name>Lp</Name><Origin><Source>GeometricFeature</Source><FeatureName>+z surface</FeatureName></Origin><PrimaryAxis><DefinedDirection>+Z</DefinedDirection><Source>ReferenceFrame</Source><SourceDirection>+Z</SourceDirection><FeatureName></FeatureName></PrimaryAxis><SecondaryAxis><DefinedDirection>+X</DefinedDirection><Source>ReferenceFrame</Source><SourceDirection>+X</SourceDirection><FeatureName></FeatureName></SecondaryAxis></Value></Frame></Frames>
  Transform Ground Center : sm_lib/Frames and Transforms/Rigid Transform  RotationMethod=None  FollAlignAxisA=+X  BaseAlignAxisA=+Y  FollAlignAxisB=+Y  BaseAlignAxisB=+Z  RotationStandardAxis=+Z  RotationAngle=0.0  RotationAngleUnits=deg  RotationArbitraryAxis=[0 0 1]  RotationSequenceAxes=FollowerAxes  RotationSequence=XYX  RotationSequenceAngles=[0 0 0]  RotationSequenceAnglesUnits=deg  RotationMatrix=[1 0 0; 0 1 0; 0 0 1]  Quaternion=[1 0 0 0]  TranslationMethod=Cartesian  TranslationCartesianOffset=[offset_x offset_y -planedepth/2]  TranslationCartesianOffsetUnits=m  TranslationStandardAxis=-Z  TranslationStandardOffset=0  TranslationStandardOffsetUnits=m  TranslationROffset=0  TranslationROffsetUnits=m  TranslationThetaOffset=0  TranslationThetaOffsetUnits=deg  TranslationZOffset=0  TranslationZOffsetUnits=m
  Lp : PMIOPort  Side=Right
  W : PMIOPort  Port=2  Side=Left
  connections:
  Lp/RConn1 -- Ground/LConn1
  Transform Ground Center/RConn1 -- Ground/RConn1
  W/RConn1 -- Transform Ground Center/LConn1

== system nonop_quadcopter_package_delivery/Quadcopter/Ground/Trajectory ==
  Spline : sm_lib/Curves and Surfaces/Spline  DataPoints=wayp_path_vis  DataPointsUnits=m  EndConditionType=Natural  GraphicType=FromGeometry  MarkerShape=Sphere  MarkerSize=10  GraphicVisPropType=SimpleVisualProperties  GraphicDiffuseColor=[1.0 1.0 0.2]  GraphicOpacity=0.5  GraphicSpecularColor=[0.5 0.5 0.5 1.0]  GraphicAmbientColor=[0.15 0.15 0.15 1.0]  GraphicEmissiveColor=[0.0 0.0 0.0 1.0]  GraphicShininess=75
  Waypoints : sm_lib/Curves and Surfaces/Point Cloud  CoordinatesMatrix=unique(waypoints','rows')  CoordinatesMatrixUnits=m  GraphicType=MarkerCloud  GraphicSphereRadius=2e-1  GraphicSphereRadiusUnits=m  GraphicVisPropType=SimpleVisualProperties  GraphicDiffuseColor=[0.302 0.7451 0.9333]  GraphicOpacity=0.5  GraphicSpecularColor=[0.5 0.5 0.5 1.0]  GraphicAmbientColor=[0.15 0.15 0.15 1.0]  GraphicEmissiveColor=[0.0 0.0 0.0 1.0]  GraphicShininess=75
  W : PMIOPort  Side=Right
  connections:
  Spline/LConn1 -- W/RConn1 -- Waypoints/LConn1
